simulink model "Euler_Moment_Equations"  (R2023a)
settings: Solver=VariableStepAuto  StartTime=0.0  StopTime=20  RelTol=1e-8
settings Model: Creator=ganes  LastModifiedBy=ganes

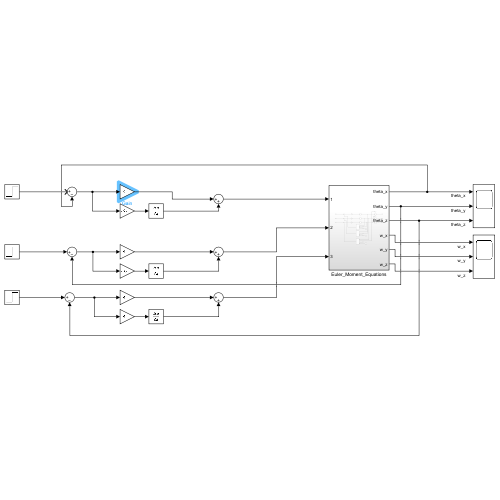
[thumbnail: Simulink's stored preview of the top-level diagram]
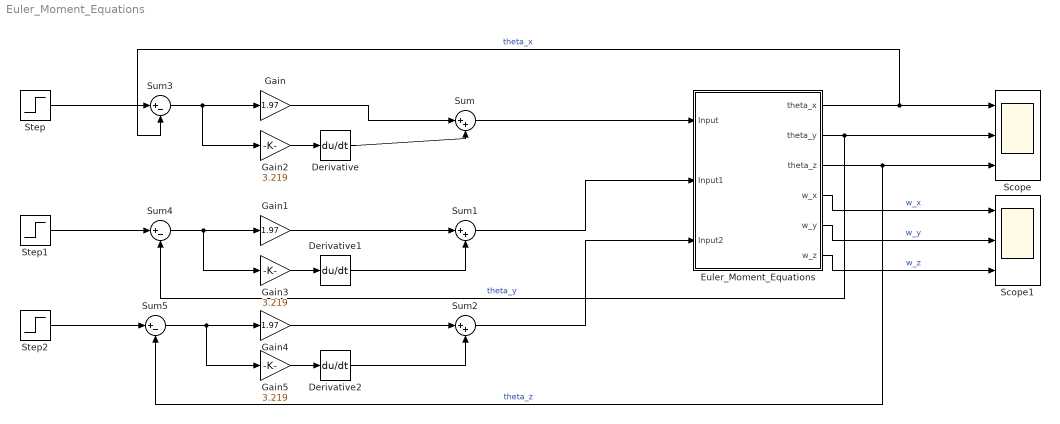
== system Euler_Moment_Equations ==
  Derivative : Derivative
  Derivative1 : Derivative
  Derivative2 : Derivative
  Euler_Moment_Equations : Subsystem
  Gain : Gain  Gain=1.97
  Gain1 : Gain  Gain=1.97
  Gain2 : Gain  Gain=3.219
  Gain3 : Gain  Gain=3.219
  Gain4 : Gain  Gain=1.97
  Gain5 : Gain  Gain=3.219
  Scope : Scope  NumInputPorts=3
  Scope1 : Scope  NumInputPorts=3
  Step : Step  Time=0  SampleTime=0
  Step1 : Step  Time=0  SampleTime=0
  Step2 : Step  Time=0  SampleTime=0
  Sum : Sum  Inputs=|++
  Sum1 : Sum  Inputs=|++
  Sum2 : Sum  Inputs=|++
  Sum3 : Sum  Inputs=|+-
  Sum4 : Sum  Inputs=|+-
  Sum5 : Sum  Inputs=|+-
  wires:
  Derivative/1 -> Sum/2
  Gain2/1 -> Derivative/1
  Gain/1 -> Sum/1
  Sum/1 -> Euler_Moment_Equations/1(Input)
  Derivative1/1 -> Sum1/2
  Gain3/1 -> Derivative1/1
  Gain1/1 -> Sum1/1
  Sum1/1 -> Euler_Moment_Equations/2(Input1)
  Derivative2/1 -> Sum2/2
  Gain5/1 -> Derivative2/1
  Gain4/1 -> Sum2/1
  Sum2/1 -> Euler_Moment_Equations/3(Input2)
  Sum3/1 -> Gain2/1, Gain/1
  Sum4/1 -> Gain3/1, Gain1/1
  Sum5/1 -> Gain5/1, Gain4/1
  Step/1 -> Sum3/1
  Step1/1 -> Sum4/1
  Step2/1 -> Sum5/1
  Euler_Moment_Equations/1(theta_x) -> Scope/1, Sum3/2  "theta_x"
  Euler_Moment_Equations/2(theta_y) -> Sum4/2, Scope/2  "theta_y"
  Euler_Moment_Equations/3(theta_z) -> Sum5/2, Scope/3  "theta_z"
  Euler_Moment_Equations/4(w_x) -> Scope1/1  "w_x"
  Euler_Moment_Equations/5(w_y) -> Scope1/2  "w_y"
  Euler_Moment_Equations/6(w_z) -> Scope1/3  "w_z"

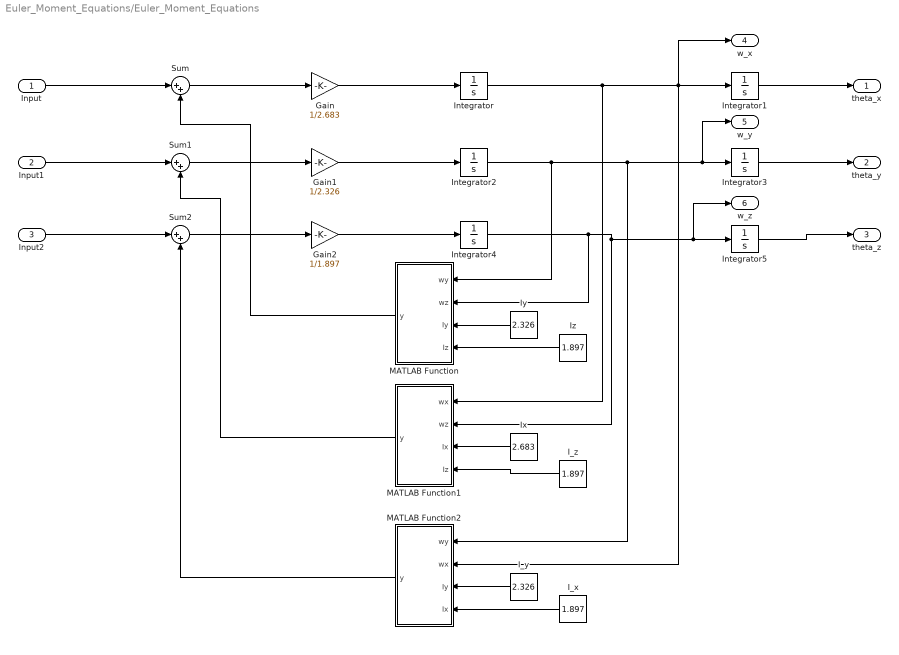
== system Euler_Moment_Equations/Euler_Moment_Equations ==
  Input : Inport
  Input1 : Inport  Port=2
  Input2 : Inport  Port=3
  Gain : Gain  Gain=1/2.683
  Gain1 : Gain  Gain=1/2.326
  Gain2 : Gain  Gain=1/1.897
  I_x : Constant  Value=1.897
  I_y : Constant  Value=2.326
  I_z : Constant  Value=1.897
  Integrator{,1..5} (6 alike) : Integrator
  Ix : Constant  Value=2.683
  Iy : Constant  Value=2.326
  Iz : Constant  Value=1.897
  MATLAB Function : MATLAB Function  TreatAsAtomicUnit=on
  MATLAB Function1 : MATLAB Function  TreatAsAtomicUnit=on
  MATLAB Function2 : MATLAB Function  TreatAsAtomicUnit=on
  Sum : Sum  Inputs=|++
  Sum1 : Sum  Inputs=|++
  Sum2 : Sum  Inputs=|++
  theta_x : Outport
  theta_y : Outport  Port=2
  theta_z : Outport  Port=3
  w_x : Outport  Port=4
  w_y : Outport  Port=5
  w_z : Outport  Port=6
  wires:
  Gain2/1 -> Integrator4/1
  Input/1 -> Sum/1
  Integrator4/1 -> MATLAB Function/2(wz), MATLAB Function1/2(wz), w_z/1, Integrator5/1
  Integrator2/1 -> MATLAB Function/1(wy), MATLAB Function2/1(wy), w_y/1, Integrator3/1
  I_y/1 -> MATLAB Function2/3(Iy)
  Iy/1 -> MATLAB Function/3(Iy)
  Sum/1 -> Gain/1
  Integrator3/1 -> theta_y/1
  Ix/1 -> MATLAB Function1/3(Ix)
  Input1/1 -> Sum1/1
  Integrator/1 -> MATLAB Function1/1(wx), w_x/1, MATLAB Function2/2(wx), Integrator1/1
  Integrator5/1 -> theta_z/1
  MATLAB Function1/1(y) -> Sum1/2
  Iz/1 -> MATLAB Function/4(Iz)
  Integrator1/1 -> theta_x/1
  I_z/1 -> MATLAB Function1/4(Iz)
  MATLAB Function/1(y) -> Sum/2
  MATLAB Function2/1(y) -> Sum2/2
  Input2/1 -> Sum2/1
  Sum2/1 -> Gain2/1
  Gain1/1 -> Integrator2/1
  Sum1/1 -> Gain1/1
  Gain/1 -> Integrator/1
  I_x/1 -> MATLAB Function2/4(Ix)

== matlab function Euler_Moment_Equations/MATLAB Function1 ==
  data: wx input; y output; wz input; Ix input; Iz input
function y = fcn(wx,wz,Ix,Iz)
y=(Ix-Iz)*wx*wz
end

== matlab function Euler_Moment_Equations/MATLAB Function ==
  data: wy input; y output; wz input; Iy input; Iz input
function y = fcn(wy,wz,Iy,Iz)
y=(Iy-Iz)*wy*wz
end

== matlab function Euler_Moment_Equations/MATLAB Function2 ==
  data: wy input; y output; wx input; Iy input; Ix input
function y = fcn(wy,wx,Iy,Ix)
y=(Iy-Ix)*wy*wx
end
